simulink model "x1sup_isolated"  (Simulink 10.3)
settings: Solver=ode45  StartTime=0.0  StopTime=10.0  RelTol=1e-3  EnableMultiTasking=on
libraries: cdsAdcx0 x1, sus_single_plant x1, cdsFilt x1, cdsParameters x1
settings Model: Creator=controls  LastModifiedBy=controls
settings DataIOCC: LimitDataPoints=on
settings OptimizationCC: InitFltsAndDblsToZero=on
settings DebuggingCC: SolverPrmCheckMsg=warning

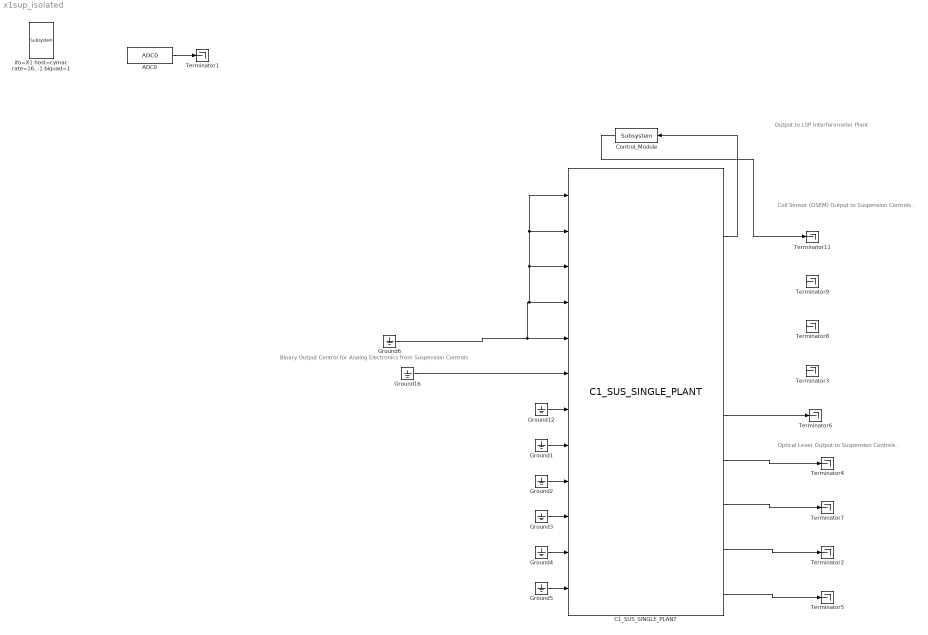
== system x1sup_isolated ==
  note: Output
      | to
      | LSP
      |                      Interferometer
      | Plant
  note: Optical
      | Lever
      | Output
      | to
      | Suspension
      | Controls
      |
      |
      |
      | .
  note: Coil
      | Sensor
      | (OSEM)
      | Output
      | to
      | Suspension
      | Controls
      |
      |
      |
      | .
  note: Binary Output
      | Control for
      | Analog
      | Electronics
      | from
      | Suspension
      | Controls
  ADC0 : cdsAdcx0/ADC0  Tag=cdsAdc  Description=|  SystemSampleTime=-1  VariantActivationTime=update diagram  Latency=0  AutoFrameSizeCalculation=off
      | type-GSC_16AI64SSA
      | card_num=0
      settings: AttributesFormatString=%<Description>\n%<Tag>
  C1_SUS_SINGLE_PLANT : sus_single_plant/C1_SUS_SINGLE_PLANT  SystemSampleTime=-1  VariantActivationTime=update diagram  Latency=0  AutoFrameSizeCalculation=off
  Control_Module : cdsFilt/Subsystem  Tag=cdsFilt  Description=|  SystemSampleTime=-1  VariantActivationTime=update diagram  Latency=0  AutoFrameSizeCalculation=off
      | Purpose:                                                                                                                                                                                                                                  
      | Standard CDS IIR filter module.                                                                                                                                                                                                           
      |                                                                                                                                                                                                                                           
      | Operation:                                                                                                                                                                                                                                
      | Consists of 10 second order section IIR filters, plus a ramped gain stage. In FE code, also provides pre-defined test points and excitation channel inputs. The filter coefficients are defined in the LIGO system using the 'foton' tool.
      |                                                                                                                                                                                                                                           
      | Usage:                                                                                                                                                                                                                                    
      | Name the part with the desired filter module name.
      settings: AttributesFormatString=%<Tag>
  Ground{1..6,12,16} (8 alike) : Ground
  Terminator{1..9,11} (10 alike) : Terminator
  ifo=X1 host=cymac rate=16K dcuid=8 specific_cpu=4 shmem_daq=1 adcSlave=1 biquad=1 : cdsParameters/Subsystem  Tag=cdsParameters  SystemSampleTime=-1  VariantActivationTime=update diagram  Latency=0  AutoFrameSizeCalculation=off
      settings: AttributesFormatString=%<Tag>
  wires:
  Ground16/1 -> C1_SUS_SINGLE_PLANT/6
  Ground1/1 -> C1_SUS_SINGLE_PLANT/8
  Ground2/1 -> C1_SUS_SINGLE_PLANT/9
  Ground3/1 -> C1_SUS_SINGLE_PLANT/10
  Ground4/1 -> C1_SUS_SINGLE_PLANT/11
  Ground5/1 -> C1_SUS_SINGLE_PLANT/12
  Ground12/1 -> C1_SUS_SINGLE_PLANT/7
  ADC0/1 -> Terminator1/1
  Ground6/1 -> C1_SUS_SINGLE_PLANT/1, C1_SUS_SINGLE_PLANT/2, C1_SUS_SINGLE_PLANT/3, C1_SUS_SINGLE_PLANT/4, C1_SUS_SINGLE_PLANT/5
  C1_SUS_SINGLE_PLANT/10 -> Terminator5/1
  C1_SUS_SINGLE_PLANT/9 -> Terminator2/1
  C1_SUS_SINGLE_PLANT/8 -> Terminator7/1
  C1_SUS_SINGLE_PLANT/7 -> Terminator4/1
  C1_SUS_SINGLE_PLANT/6 -> Terminator6/1
  C1_SUS_SINGLE_PLANT/2 -> Control_Module/1
  Control_Module/1 -> Terminator11/1
